simulink model "esercizioS"  (R2020a)
settings: Solver=VariableStepAuto  StartTime=0.0  StopTime=10.0  RelTol=1e-3
values from neighbouring files (symbols this model uses):
  A = -5    [esempio0.m]    (also in esercizio.m = [-1 -2; 1 -1]; esercizio2.m = [0 2; -10 -12]; esercizio3.m = [0 1; -5 -1]; esercizio4.m = [-7 1; -12 0])
  Ahat = A-B*K    [esempio0.m]    (also in esercizio.m; esercizio2.m; esercizio3.m; esercizio4.m)
  B = 1    [esempio0.m]    (also in esercizio.m = [0;1]; esercizio2.m = [0;1]; esercizio3.m = [0;1]; esercizio4.m = [0;1])
  C = 1    [esempio0.m]    (also in esercizio.m = [1 0;0 1]; esercizio2.m = [1 0;0 1]; esercizio3.m = [1 0; 0 1]; esercizio4.m = [1 0; 0 1])
  D = 0    [esempio0.m]    (also in esercizio.m = zeros(2,1); esercizio2.m = zeros(2,1); esercizio3.m = zeros(2,1); esercizio4.m = zeros(2,1))
  K = place(A, B, P)    [esempio0.m]    (also in esercizio.m; esercizio2.m; esercizio3.m; esercizio4.m)
settings Model: Creator=itama  LastModifiedBy=itama

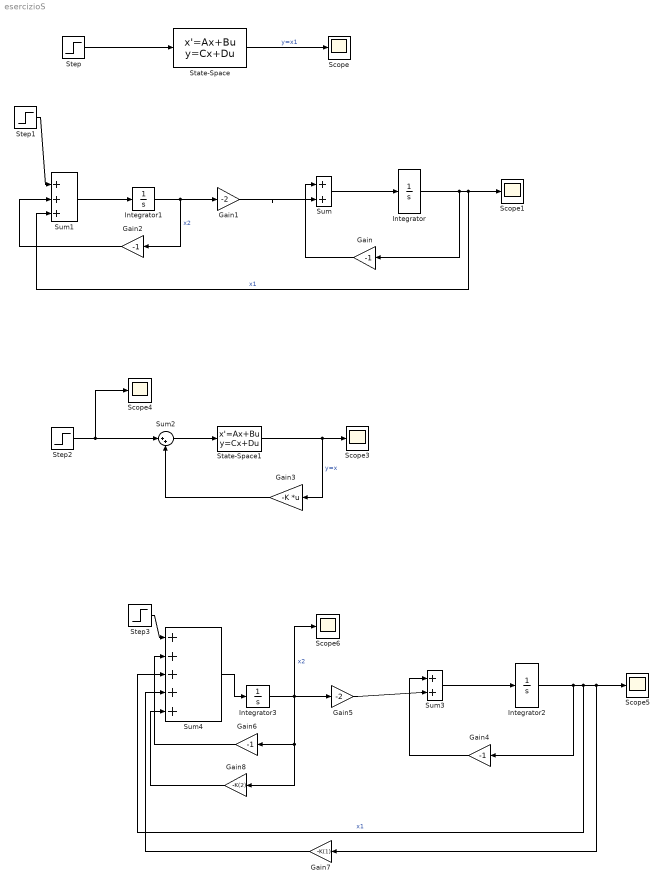
== system esercizioS ==
  Gain{,2,4,6} (4 alike) : Gain  Gain=-1
  Gain1 : Gain  Gain=-2
  Gain3 : Gain  Gain=-K  Multiplication=Matrix(K*u)
  Gain5 : Gain  Gain=-2
  Gain7 : Gain  Gain=-K(1)
  Gain8 : Gain  Gain=-K(2)
  Integrator{,1..3} (4 alike) : Integrator
  Scope{,1,3..6} (6 alike) : Scope
  State-Space : StateSpace  A=A  B=B  C=C  D=D  InitialCondition=[0;0]
  State-Space1 : StateSpace  A=Ahat  B=B  C=C  D=D  InitialCondition=[0;0]
  Step{,1..3} (4 alike) : Step  SampleTime=0
  Sum : Sum  Inputs=|++
  Sum1 : Sum  Inputs=|+++
  Sum2 : Sum  Inputs=|++
  Sum3 : Sum  Inputs=|++
  Sum4 : Sum  Inputs=|+++++
  wires:
  State-Space/1 -> Scope/1  "y=x1"
  Step/1 -> State-Space/1
  Integrator/1 -> Gain/1, Scope1/1, Sum1/3  "x1"
  Gain/1 -> Sum/1
  Gain1/1 -> Sum/2
  Integrator1/1 -> Gain2/1, Gain1/1  "x2"
  Step1/1 -> Sum1/1
  Gain2/1 -> Sum1/2
  Sum1/1 -> Integrator1/1
  Sum/1 -> Integrator/1
  Step2/1 -> Scope4/1, Sum2/1
  Sum2/1 -> State-Space1/1
  Gain3/1 -> Sum2/2
  State-Space1/1 -> Gain3/1, Scope3/1  "y=x"
  Gain6/1 -> Sum4/2
  Sum4/1 -> Integrator3/1
  Step3/1 -> Sum4/1
  Integrator3/1 -> Gain8/1, Gain6/1, Scope6/1, Gain5/1  "x2"
  Gain4/1 -> Sum3/1
  Gain5/1 -> Sum3/2
  Sum3/1 -> Integrator2/1
  Integrator2/1 -> Gain4/1, Sum4/3, Gain7/1, Scope5/1  "x1"
  Gain7/1 -> Sum4/4
  Gain8/1 -> Sum4/5
